simulink model "hw12"  (R2018a)
settings: Solver=VariableStepAuto  StartTime=0.0  StopTime=50.0  FixedStep=0.01  RelTol=1e-3
values from neighbouring files (symbols this model uses):
  a = b/m    (= 2)    [HW1_1.m]    (also in HW1_12.m = 0.2)
  c = k/m    (= 1)    [HW1_1.m]    (also in HW1_12.m)
  d = 1/m    (= 1)    [HW1_1.m]    (also in HW1_12.m)
  X = 0    [HW1_12.m]
  Y = 1    [HW1_12.m]
settings Model: Creator=labuser  LastModifiedBy=Halil Temurtaş
settings CodeAppCC: StateflowObjectComments=on

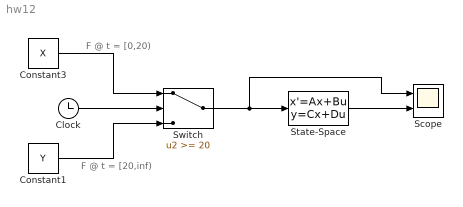
== system hw12 ==
  note: F @ t = [0,20)
  note: F @ t = [20,inf)
  Clock : Clock
  Constant1 : Constant  Value=Y
  Constant3 : Constant  Value=X
  Scope : Scope  NumInputPorts=2
  State-Space : StateSpace  A=[0 1; -a -c]  B=[0 ; d]  C=[1 0]  D=[0]  InitialCondition=0  ContinuousStateAttributes={'position','velocity'}
  Switch : Switch  Threshold=20
  wires:
  State-Space/1 -> Scope/2
  Clock/1 -> Switch/2
  Constant3/1 -> Switch/1
  Constant1/1 -> Switch/3
  Switch/1 -> Scope/1, State-Space/1
